simulink model "BackStepping"  (R2018b)
settings: Solver=FixedStepAuto  StartTime=0.0  StopTime=10  FixedStep=0.001  RelTol=1e-3  EnableMultiTasking=on
InitFcn:
  | X0 = randn(1)*10 ;
settings Model: Creator=omid_zandi  LastModifiedBy=Arash
settings OptimizationCC: LifeSpan=inf
settings DebuggingCC: SFUnexpectedBacktrackingDiag=warning  SFNoUnconditionalDefaultTransitionDiag=warning
settings SFSimCC: SimUseLocalCustomCode=off
settings RTWCC: RTWUseLocalCustomCode=off
settings CodeAppCC: StateflowObjectComments=on
settings GRTTargetCC: TargetLangStandard=C89/C90 (ANSI)  GeneratePreprocessorConditionals=Disable all
settings ConfigComp: CovMetricSettings=dw  CovHtmlReporting=on  CovSaveCumulativeToWorkspaceVar=on  CovSaveSingleToWorkspaceVar=on  CovExternalEMLEnable=off

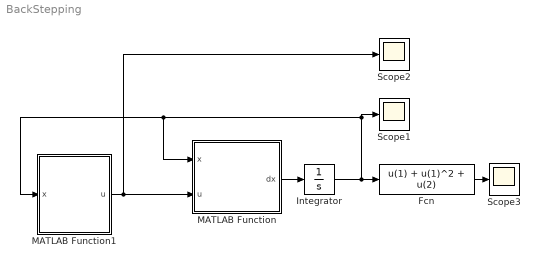
== system BackStepping ==
  Fcn : Fcn  Expr=u(1) + u(1)^2 + u(2)
  Integrator : Integrator  InitialCondition=randn(2,1)
  MATLAB Function : MATLAB Function  TreatAsAtomicUnit=on
  MATLAB Function1 : MATLAB Function  TreatAsAtomicUnit=on
  Scope1 : Scope
  Scope2 : Scope
  Scope3 : Scope
  wires:
  MATLAB Function/1(dx) -> Integrator/1
  MATLAB Function1/1(u) -> MATLAB Function/2(u), Scope2/1
  Integrator/1 -> Fcn/1, Scope1/1, MATLAB Function1/1(x), MATLAB Function/1(x)
  Fcn/1 -> Scope3/1

== matlab function BackStepping/MATLAB Function1 ==
  data: x input; u output
function u = fcn(x )
u  =-(x(1) + x(2) + (x(1)^2 + x(2))*(2 * x(1) + 1))-(x(1) + x(2) + x(1)^2) ;

== matlab function BackStepping/MATLAB Function ==
  data: x input; u input; dx output
function dx = fcn(x  ,u)
dx = zeros(2,1) ;
dx(1) = x(1)^2 + x(2);
dx(2) = x(2) + u ;
